simulink model "Create_4x4_Matrix"  (R2017a)
settings: Solver=VariableStepAuto  StartTime=0.0  StopTime=10.0  RelTol=1e-3
settings Model: Creator=tlum1  LastModifiedBy=tlum1

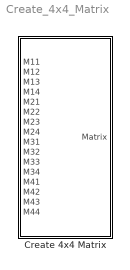
== system Create_4x4_Matrix ==
  Create 4x4 Matrix : Subsystem

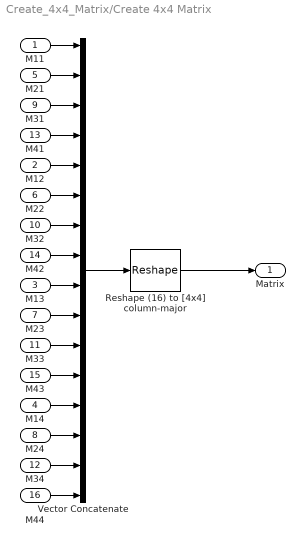
== system Create_4x4_Matrix/Create 4x4 Matrix ==
  M11 : Inport  PortDimensions=1
  M12 : Inport  Port=2  PortDimensions=1
  M13 : Inport  Port=3  PortDimensions=1
  M14 : Inport  Port=4  PortDimensions=1
  M21 : Inport  Port=5  PortDimensions=1
  M22 : Inport  Port=6  PortDimensions=1
  M23 : Inport  Port=7  PortDimensions=1
  M24 : Inport  Port=8  PortDimensions=1
  M31 : Inport  Port=9  PortDimensions=1
  M32 : Inport  Port=10  PortDimensions=1
  M33 : Inport  Port=11  PortDimensions=1
  M34 : Inport  Port=12  PortDimensions=1
  M41 : Inport  Port=13  PortDimensions=1
  M42 : Inport  Port=14  PortDimensions=1
  M43 : Inport  Port=15  PortDimensions=1
  "M44 " : Inport  Port=16  PortDimensions=1
  Reshape (16) to [4x4] column-major : Reshape  OutputDimensionality=Customize  OutputDimensions=[4,4]
  Vector Concatenate : Concatenate  NumInputs=16
  Matrix : Outport
  wires:
  M41/1 -> Vector Concatenate/4
  M23/1 -> Vector Concatenate/10
  M42/1 -> Vector Concatenate/8
  M33/1 -> Vector Concatenate/11
  M31/1 -> Vector Concatenate/3
  Vector Concatenate/1 -> Reshape (16) to [4x4] column-major/1
  M24/1 -> Vector Concatenate/14
  M21/1 -> Vector Concatenate/2
  M12/1 -> Vector Concatenate/5
  "M44 "/1 -> Vector Concatenate/16
  M22/1 -> Vector Concatenate/6
  M34/1 -> Vector Concatenate/15
  M11/1 -> Vector Concatenate/1
  M14/1 -> Vector Concatenate/13
  M43/1 -> Vector Concatenate/12
  M13/1 -> Vector Concatenate/9
  M32/1 -> Vector Concatenate/7
  Reshape (16) to [4x4] column-major/1 -> Matrix/1
